simulink model "lindiscrmodel_obs_report"  (R2019a)
settings: Solver=VariableStepAuto  StartTime=0.0  StopTime=20  RelTol=1e-3
InitFcn:
  | lindiscrmodel
values from neighbouring files (symbols this model uses):
  L1 = place(linmat.A1',linmat.C1',pdes1)'    [lindiscrmodel.m]
  linmat =     [linmat_sim.mat]
  R_kal = cov(theta.data)    [lindiscrmodel.m]
  Ts = 0.01    [lindiscrmodel.m]
undefined symbols (not defined in the file or in its folder): Discrete, Time
libraries: ctrlSharedLib x1
settings Model: Creator=jessi  LastModifiedBy=jessi

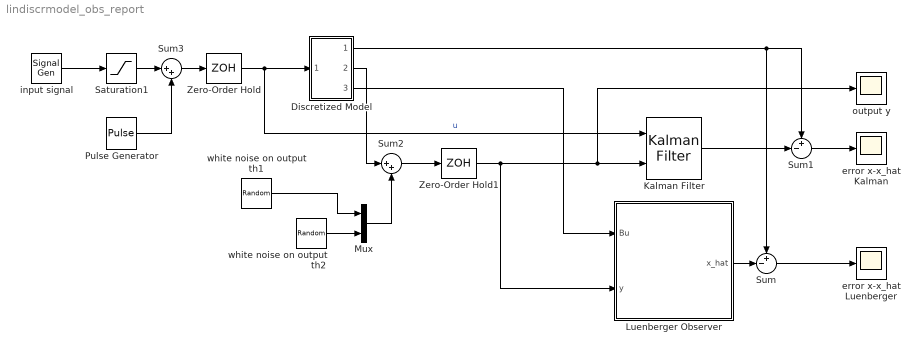
== system lindiscrmodel_obs_report ==
  Discretized Model : Subsystem
  Kalman Filter : ctrlSharedLib/Kalman Filter  TimeDomain=Discrete-Time  UseCurrentEstimator=on  ModelSource=Individual A, B, C, D matrices  ModelSourceVariable=sysd2  A=linmat.A1  B=linmat.B1  C=linmat.C1  D=linmat.D1  NumberOfStates=1  NumberOfInputs=1  NumberOfOutputs=1  InitialEstimateSource=Dialog  X0=[0;0;0;0]  P0=10  UseK=off  UseGH=off  NumberOfProcessNoiseInputs=1  G=1  TimeInvariantG=on  H=0  TimeInvariantH=on  Q=0.000001*diag([1 1 1 1])  TimeInvariantQ=on  R=R_kal  TimeInvariantR=on  N=0  TimeInvariantN=on  AddInputPort=on  AddEnablePort=off  OutputEstimatedY=off  OutputP=off  Ts=Ts
      settings: SourceProductBaseCode=CT
  Luenberger Observer : Subsystem
  Mux : Mux  Inputs=2
  Pulse Generator : DiscretePulseGenerator  PulseType=Time based  Amplitude=0.5  Period=5  PulseWidth=5
  Saturation1 : Saturate  UpperLimit=1  LowerLimit=-1
  Sum : Sum  Inputs=+-|
  Sum1 : Sum  Inputs=+-|
  Sum2 : Sum  Inputs=|++
  Sum3 : Sum  Inputs=|++
  Zero-Order Hold : ZeroOrderHold  SampleTime=Ts
  Zero-Order Hold1 : ZeroOrderHold  SampleTime=Ts
  error x-x_hat Kalman : Scope
  error x-x_hat Luenberger : Scope
  input signal : SignalGenerator  Amplitude=0
  output y : Scope
  white noise on output th1 : RandomNumber  Variance=0.00001  SampleTime=0.01
  white noise on output th2 : RandomNumber  Variance=0.00001  SampleTime=0.01
  wires:
  input signal/1 -> Saturation1/1
  Sum3/1 -> Zero-Order Hold/1
  Saturation1/1 -> Sum3/1
  Zero-Order Hold/1 -> Discretized Model/1(u[k]), Kalman Filter/1  "u"
  Sum2/1 -> Zero-Order Hold1/1
  Zero-Order Hold1/1 -> Luenberger Observer/2(y), output y/1, Kalman Filter/2
  Mux/1 -> Sum2/2
  white noise on output th2/1 -> Mux/2
  white noise on output th1/1 -> Mux/1
  Sum/1 -> error x-x_hat Luenberger/1
  Kalman Filter/1 -> Sum1/2
  Luenberger Observer/1(x_hat) -> Sum/2
  Discretized Model/3(Bu[k]) -> Luenberger Observer/1(Bu)
  Discretized Model/1(x[k]) -> Sum1/1, Sum/1
  Discretized Model/2(y[k]) -> Sum2/1
  Pulse Generator/1 -> Sum3/2
  Sum1/1 -> error x-x_hat Kalman/1

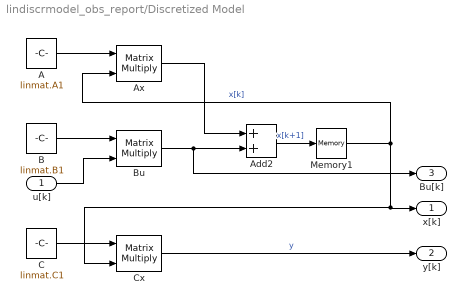
== system lindiscrmodel_obs_report/Discretized Model ==
  u[k] : Inport
  A : Constant  Value=linmat.A1  SampleTime=Ts
  Add2 : Sum
  Ax : Product  Multiplication=Matrix(*)
  B : Constant  Value=linmat.B1  SampleTime=Ts
  Bu : Product  Multiplication=Matrix(*)
  C : Constant  Value=linmat.C1  SampleTime=Ts
  Cx : Product  Multiplication=Matrix(*)
  Memory1 : Memory  InitialCondition=[0;0;0;0]
  x[k] : Outport
  y[k] : Outport  Port=2
  Bu[k] : Outport  Port=3
  wires:
  B/1 -> Bu/1
  Memory1/1 -> x[k]/1, Cx/2, Ax/2  "x[k]"
  Add2/1 -> Memory1/1  "x[k+1]"
  C/1 -> Cx/1
  A/1 -> Ax/1
  u[k]/1 -> Bu/2
  Ax/1 -> Add2/1
  Bu/1 -> Bu[k]/1, Add2/2
  Cx/1 -> y[k]/1  "y"

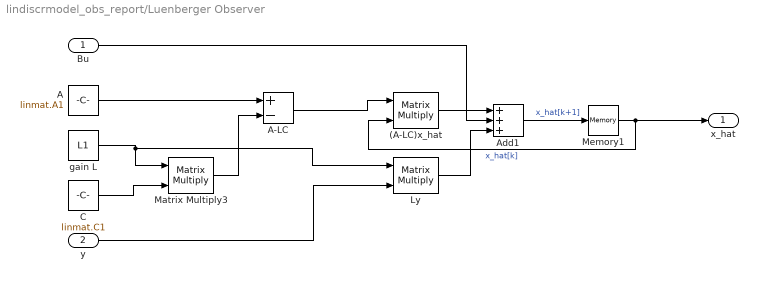
== system lindiscrmodel_obs_report/Luenberger Observer ==
  Bu : Inport
  y : Inport  Port=2
  (A-LC)x_hat : Product  Multiplication=Matrix(*)
  A : Constant  Value=linmat.A1  SampleTime=Ts
  A-LC : Sum  Inputs=+-
  Add1 : Sum  Inputs=+++
  C : Constant  Value=linmat.C1  SampleTime=Ts
  Ly : Product  Multiplication=Matrix(*)
  Matrix Multiply3 : Product  Multiplication=Matrix(*)
  Memory1 : Memory  InitialCondition=[0;0;0;0]
  gain L : Constant  Value=L1  SampleTime=Ts
  x_hat : Outport
  wires:
  gain L/1 -> Matrix Multiply3/1, Ly/1
  Ly/1 -> Add1/3
  C/1 -> Matrix Multiply3/2
  A/1 -> A-LC/1
  Bu/1 -> Add1/2
  Add1/1 -> Memory1/1  "x_hat[k+1]"
  Matrix Multiply3/1 -> A-LC/2
  A-LC/1 -> (A-LC)x_hat/1
  (A-LC)x_hat/1 -> Add1/1
  Memory1/1 -> x_hat/1, (A-LC)x_hat/2  "x_hat[k]"
  y/1 -> Ly/2
